simulink model "EE463_complete_term_project"  (R2020b)
settings: Solver=FixedStepDiscrete  StartTime=0.0  StopTime=5  FixedStep=1e-07  RelTol=1e-3
undefined symbols (not defined in the file): Acid, Lead, Ts
libraries: powerlib x26, powerlib_meascontrol x3, electricdrivelib x1, pid_lib x1
settings Model: SimulationMode=accelerator  Creator=ayaz  LastModifiedBy=mehme
settings SFSimCC: CustomCodeUndefinedFunction=UseInterfaceOnly

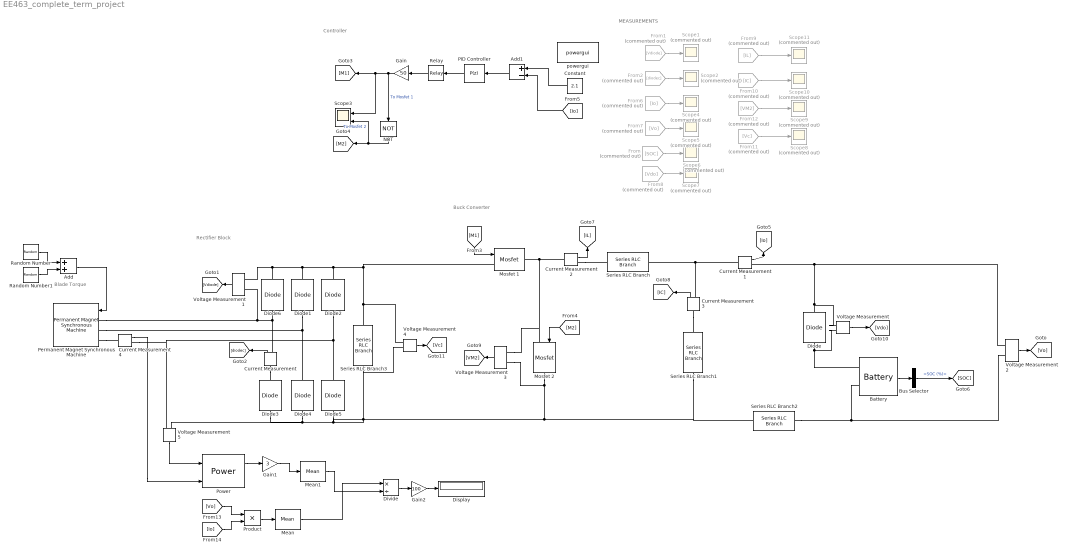
== system EE463_complete_term_project ==
  note: MEASUREMENTS
  note: Controller
  note: Buck Converter
  note: Blade Torque
  note: Rectifier Block
  Add : Sum
  Add1 : Sum  Inputs=+-
  Battery : electricdrivelib/Extra Sources/Battery  BatType=Lead-Acid  ShowTempParam=off  ThermalPreset=no  ShowAgeParam=off  NomV=24  NomQ=13  SOC=50  Batt_Tr=30  PresetModel=on  MaxQ=13.5417  MinV=18  FullV=26.1316  Dis_rate=2.6  R=0.018462  Normal_OP=4.0336  expZone="[24.4342    0.0433333]"  current=[6.5 13 32.5]  Units=Time  Tci=20  NomT=20  T2=-30  MaxQ2=4.8  FullV2=7.1  Normal_OP2=5.655  expZone2="[6.58           1]"  Rca=0.6  ti=2000  Dp=0  Neq0=0  Tsim=1e6  Ta1=25  Qeol=5.4*0.9  Reol=0.013333*1.2  Char_age=[2.3478, 3]  Dis_age=[2.3478, 10]  N1=1500  N2=10500  N3=1000  N4=1400  Ta2=45  N5=950
  Bus Selector : BusSelector  OutputSignals=SOC (%)
  Constant : Constant  Value=2.1
  Current Measurement{,1..4} (5 alike) : powerlib/Measurements/Current Measurement  PhasorSimulation=off  OutputType=Complex  PSBequivalent=0
  Diode : powerlib/Power Electronics/Diode  Ron=0.001  Lon=0  Vf=0.8  IC=0  UseSnubber=0  Rs=500000  Cs=250e-11  Measurements=off
  Diode{1..6} (6 alike) : powerlib/Power Electronics/Diode  Ron=Ron  Lon=0  Vf=Vfmax  IC=0  UseSnubber=off  Rs=50000  Cs=250e-11  Measurements=off
  Display : Display
  Divide : Product  Inputs=*/
  From : From  Commented=on  GotoTag=SOC
  From1 : From  Commented=on  GotoTag=Vdiode
  From10 : From  Commented=on  GotoTag=IC
  From11 : From  Commented=on  GotoTag=Vc
  From12 : From  Commented=on  GotoTag=VM2
  From2 : From  Commented=on  GotoTag=diodec
  From6 : From  Commented=on  GotoTag=Io
  From7 : From  Commented=on  GotoTag=Vo
  From8 : From  Commented=on  GotoTag=Vdo
  From9 : From  Commented=on  GotoTag=IL
  Gain : Gain  Gain=50
  Gain1 : Gain  Gain=3
  Gain2 : Gain  Gain=100
  Mean : powerlib_meascontrol/Measurements/Mean  Freq=50  Vinit=0  Ts=Ts
  Mean1 : powerlib_meascontrol/Measurements/Mean  Freq=50  Vinit=0  Ts=Ts
  Mosfet 1 : powerlib/Power Electronics/Mosfet  Ron=1  Lon=0  Rd=0.01  Vfd=0  IC=0  Rs=1e5  Cs=inf  Measurements=off
  Mosfet 2 : powerlib/Power Electronics/Mosfet  Ron=0.054  Lon=0  Rd=0.01  Vfd=0  IC=0  Rs=1e5  Cs=inf  Measurements=off
  NOT : Logic  Operator=NOT  IconShape=distinctive  AllPortsSameDT=off  OutDataTypeStr=boolean
  PID Controller : pid_lib/PID Controller  Controller=P  Form=Parallel  TimeDomain=Discrete-time  UseExternalTs=off  SampleTime=Ts  IntegratorMethod=Forward Euler  FilterMethod=Forward Euler  ControllerParametersSource=internal  P=1  I=0.25  D=0  UseFilter=on  N=100  TunerSelectOption=Transfer Function Based (PID Tuner App)  InitialConditionSource=internal  InitialConditionForIntegrator=0  InitialConditionForFilter=0  DifferentiatorICPrevScaledInput=0  ExternalReset=none  TrackingMode=off  Kt=1  LimitOutput=off  SatLimitsSource=internal  UpperSaturationLimit=inf  LowerSaturationLimit=-inf  LinearizeAsGain=on  AntiWindupMode=none  Kb=1  POutMin=[]  POutMax=[]  IOutMin=[]  IOutMax=[]  DOutMin=[]  DOutMax=[]  NOutMin=[]  NOutMax=[]  SumOutMin=[]  SumOutMax=[]  SaturationOutMin=[]  SaturationOutMax=[]  PParamMin=[]  PParamMax=[]  IParamMin=[]  IParamMax=[]  DParamMin=[]  DParamMax=[]  NParamMin=[]  NParamMax=[]  KbParamMin=[]  KbParamMax=[]  KtParamMin=[]  KtParamMax=[]  KbOutMin=[]  KbOutMax=[]  KtOutMin=[]  KtOutMax=[]  IntegratorOutMin=[]  IntegratorOutMax=[]  FilterOutMin=[]  FilterOutMax=[]  SumI1OutMin=[]  SumI1OutMax=[]  SumI2OutMin=[]  SumI2OutMax=[]  SumI3OutMin=[]  SumI3OutMax=[]  SumI4OutMin=[]  SumI4OutMax=[]  SumDOutMin=[]  SumDOutMax=[]  DifferentiatorOutMin=[]  DifferentiatorOutMax=[]  FilterDiffOutCoefMin=[]  FilterDiffOutCoefMax=[]  ReciprocalOutMin=[]  ReciprocalOutMax=[]  SumDenOutMin=[]  SumDenOutMax=[]  SumNumOutMin=[]  SumNumOutMax=[]  DivideOutMin=[]  DivideOutMax=[]  UdiffTsProdOutMin=[]  UdiffTsProdOutMax=[]  NTsProdOutMin=[]  NTsProdOutMax=[]  UintegralTsProdOutMin=[]  UintegralTsProdOutMax=[]  UngainTsProdOutMin=[]  UngainTsProdOutMax=[]  IntegratorContinuousStateAttributes=''  IntegratorStateMustResolveToSignalObject=off  IntegratorRTWStateStorageClass=Auto  FilterContinuousStateAttributes=''  FilterStateMustResolveToSignalObject=off  FilterRTWStateStorageClass=Auto  ParallelPVariant=InternalParameters  IdealPVariant=Disabled  IVariant=Disabled  DVariant=Disabled  IntegratorVariant=Disabled  SatVariant=Disabled  AWVariant=Disabled  PCopyVariant=Disabled  TRVariant=Disabled  FdbkBlocksVariant=Forward  IdealPFdbkVariant=Disabled  SatFdbkVariant=Disabled  DerivativeFilterVariant=Disabled  NVariant=Disabled  NCopyVariant=Disabled_SignalSpec  FilterICVariant=Disabled  IntegratorICVariant=Disabled  ExternalResetVariant=Disabled  TRSumVariant=Passthrough  SumFdbkVariant=Disabled  SumVariant=Passthrough_P  TsampFilterVariant=InternalTs  TsampNgainVariant=Passthrough  TsampIntegralVariant=Disabled_SignalSpec  ExternalSaturationOutDataTypeStr=Inherit: Same as second input
  Permanent Magnet Synchronous Machine : powerlib/Machines/Permanent Magnet Synchronous Machine  NbPhases=3  FluxDistribution=Sinusoidal  RotorType=Round  MechanicalLoad=Torque Tm  PresetModel=No  ShowDetailedParameters=on  MeasurementBus=off  Resistance=10.58  Inductance=8.5e-3  dqInductances=[8.5e-3,8.5e-3]  La=0.0167  MachineConstant=Voltage Constant (V_peak L-L / krpm)  Flux=0.60646  VoltageCst=110  TorqueCst=0.90969  Flat=120  Mechanical=[0.00027 0.005024 1 0]  PolePairs=4  InitialConditions=[300,0, 0,0]  InitialConditions5ph=[0 0 0 0 0 0]  RefAngle=90 degrees behind phase A axis (modified Park)  IterativeDiscreteModel=Trapezoidal non iterative  TsBlock=Ts  TsPowergui=0
  Power : powerlib_meascontrol/Measurements/Power  Freq=50  Vinit=[1, 0]  Iinit=[1, 0]  Ts=Ts
  Product : Product
  Random Number : RandomNumber  Mean=-1.6  Variance=0.05  SampleTime=1
  Random Number1 : RandomNumber  Variance=0.1  SampleTime=1e-3
  Relay : Relay  OnSwitchValue=0.2  OffSwitchValue=0
  Scope{1..2,4..11} (10 alike) : Scope  Commented=on
  Scope3 : Scope  NumInputPorts=2
  Series RLC Branch : powerlib/Elements/Series RLC Branch  LConnTagsString=__new0  RConnTagsString=__new0  BranchType=RL  Resistance=1  Inductance=10e-4  SetiL0=off  InitialCurrent=0  Capacitance=1e-6  Setx0=off  InitialVoltage=0  Measurements=None
  Series RLC Branch1 : powerlib/Elements/Series RLC Branch  LConnTagsString=__new0  RConnTagsString=__new0  BranchType=C  Resistance=1  Inductance=1e-3  SetiL0=off  InitialCurrent=0  Capacitance=1.5e-6  Setx0=off  InitialVoltage=0  Measurements=None
  Series RLC Branch2 : powerlib/Elements/Series RLC Branch  LConnTagsString=__new0  RConnTagsString=__new0  BranchType=R  Resistance=0.1  Inductance=1e-3  SetiL0=off  InitialCurrent=0  Capacitance=1e-6  Setx0=off  InitialVoltage=0  Measurements=None
  Series RLC Branch3 : powerlib/Elements/Series RLC Branch  LConnTagsString=__new0  RConnTagsString=__new0  BranchType=RC  Resistance=0  Inductance=1e-3  SetiL0=off  InitialCurrent=0  Capacitance=540e-6  Setx0=off  InitialVoltage=0  Measurements=None
  Voltage Measurement{,1..5} (6 alike) : powerlib/Measurements/Voltage Measurement  PhasorSimulation=off  OutputType=Complex  PSBequivalent=0
  powergui : powerlib/powergui  Priority=1  SimulationMode=Discrete  SampleTime=Ts  frequency=60  Iterations=50  frequencyindice=0  Pbase=100e6  ErrMax=1e-4  UnitsV=kV  UnitsW=MW  buscounter=0  FunctionMessages=off  echomessages=off  EnableUseOfTLC=off  CurrentSourceSwitches=off  DisableSnubberDevices=off  DisableRonSwitches=off  DisableVfSwitches=off  DisplayEquations=off  AutomaticDiscreteSolvers=off  SolverType=Tustin/Backward Euler (TBE)  Interpol=off  ExternalGateDelay=off  methode=off  Ts=100  x0status=blocks  SPID=on  SwTol=0  HookPort=off  NonlinearTolerance=0  nMaxIteration=15  ContinueOnMaxIteration=off  RestoreLinks=warning  ResistiveCurrentMeasurement=off  Frange=[0:2:500]  Ylog=off  Xlog=on  ShowGrid=off  save=off  variable=ZData  structure=0  ZoomFFT=off  StartTime=0.0  cycles=1  DisplayStyle=1  fundamental=60  FreqAxis=off  MaxFrequency=1000  frequencyindicesteady=1  RmsSteady=1  display=off
  wires:
  Random Number/1 -> Add/1
  Random Number1/1 -> Add/2
  Add/1 -> Permanent Magnet Synchronous Machine/1
  Voltage Measurement1/1 -> [Vdiode]
  From1/1 -> Scope1/1
  Current Measurement/1 -> [diodec]
  From2/1 -> Scope2/1
  Voltage Measurement2/1 -> [Vo]
  PID Controller/1 -> Relay/1
  Add1/1 -> PID Controller/1
  Constant/1 -> Add1/1
  Gain/1 -> [M1], Scope3/1, NOT/1  "To Mosfet 1"
  Current Measurement2/1 -> [IL]
  Current Measurement3/1 -> [IC]
  Voltage Measurement3/1 -> [VM2]
  Battery/1 -> Bus Selector/1
  Bus Selector/1 -> [SOC]  "<SOC (%)>"
  [M1] -> Mosfet 1/1
  NOT/1 -> Scope3/2, [M2]  "To Mosfet 2"
  [M2] -> Mosfet 2/1
  Current Measurement1/1 -> [Io]
  [Io] -> Add1/2
  From6/1 -> Scope4/1
  From7/1 -> Scope5/1
  From/1 -> Scope6/1
  Voltage Measurement/1 -> [Vdo]
  From8/1 -> Scope7/1
  From9/1 -> Scope11/1
  From10/1 -> Scope10/1
  From12/1 -> Scope9/1
  Relay/1 -> Gain/1
  Voltage Measurement4/1 -> [Vc]
  From11/1 -> Scope8/1
  Current Measurement4/1 -> Power/2
  Voltage Measurement5/1 -> Power/1
  [Vo] -> Product/1
  [Io] -> Product/2
  Power/1 -> Gain1/1
  Product/1 -> Mean/1
  Gain1/1 -> Mean1/1
  Divide/1 -> Gain2/1
  Gain2/1 -> Display/1
  Mean/1 -> Divide/1
  Mean1/1 -> Divide/2
  connections:
  Series RLC Branch3/LConn1 -- Diode2/RConn1 -- Diode1/RConn1 -- Voltage Measurement1/LConn1 -- Diode6/RConn1 -- Mosfet 1/LConn1 -- Voltage Measurement4/LConn1
  Permanent Magnet Synchronous Machine/LConn1 -- Voltage Measurement1/LConn2 -- Current Measurement/RConn1 -- Diode6/LConn1
  Diode2/LConn1 -- Current Measurement4/RConn1 -- Voltage Measurement5/LConn1 -- Diode5/RConn1
  Diode1/LConn1 -- Permanent Magnet Synchronous Machine/LConn2 -- Diode4/RConn1
  Current Measurement/LConn1 -- Diode3/RConn1
  Current Measurement2/LConn1 -- Voltage Measurement3/LConn1 -- Mosfet 2/LConn1 -- Mosfet 1/RConn1
  Diode/LConn1 -- Current Measurement1/RConn1 -- Voltage Measurement2/LConn1 -- Voltage Measurement/LConn1
  Current Measurement1/LConn1 -- Current Measurement3/RConn1 -- Series RLC Branch/RConn1
  Current Measurement2/RConn1 -- Series RLC Branch/LConn1
  Current Measurement3/LConn1 -- Series RLC Branch1/LConn1
  Diode/RConn1 -- Battery/LConn1 -- Voltage Measurement/LConn2
  Series RLC Branch2/LConn1 -- Battery/LConn2 -- Voltage Measurement2/LConn2
  Voltage Measurement3/LConn2 -- Voltage Measurement4/LConn2 -- Series RLC Branch3/RConn1 -- Diode3/LConn1 -- Voltage Measurement5/LConn2 -- Diode4/LConn1 -- Diode5/LConn1 -- Series RLC Branch2/RConn1 -- Series RLC Branch1/RConn1 -- Mosfet 2/RConn1
  Permanent Magnet Synchronous Machine/LConn3 -- Current Measurement4/LConn1
